simulink model "MRC_OutputMeasurement"  (R2016b)
settings: Solver=VariableStepAuto  StartTime=0.0  StopTime=10.0  RelTol=1e-3
undefined symbols (not defined in the file or in its folder): sigbuilder_block
settings Model: Creator=Niels  LastModifiedBy=Niels

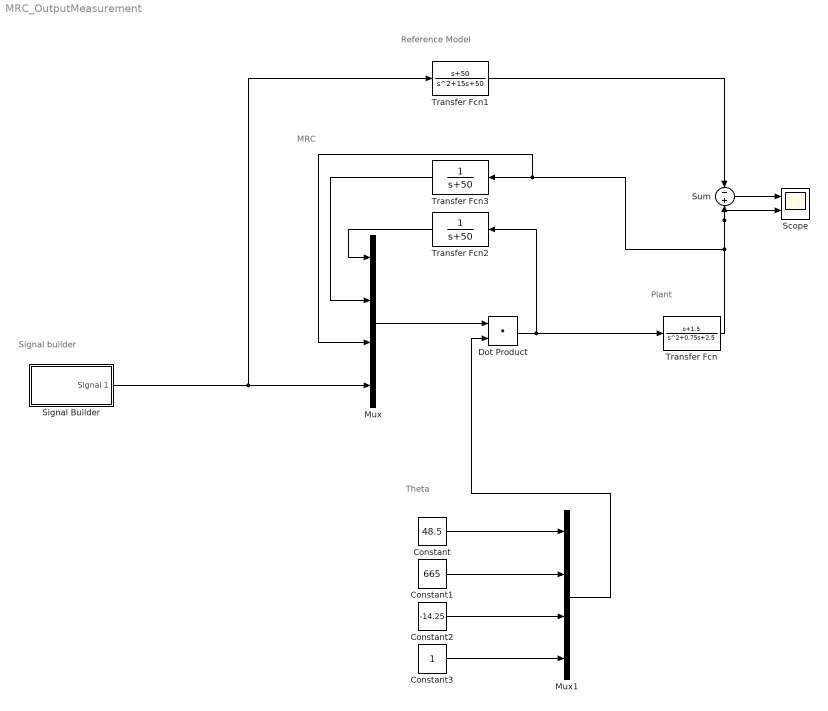
== system MRC_OutputMeasurement ==
  note: Signal builder
  note: Theta
  note: MRC
  note: Plant
  note: Reference Model
  Constant : Constant  Value=48.5
  Constant1 : Constant  Value=665
  Constant2 : Constant  Value=-14.25
  Constant3 : Constant
  Dot Product : DotProduct  InputSameDT=on  OutDataTypeStr=Inherit: Inherit via internal rule
  Mux : Mux
  Mux1 : Mux
  Scope : Scope  NumInputPorts=2
  Signal Builder : Subsystem  Tag=STV Subsys  LoadFcn=sigbuilder_block('load');  StartFcn=sigbuilder_block('start');  StopFcn=sigbuilder_block('stop');  ClipboardFcn=sigbuilder_block('clipboard');  mask(Sigbuilder block){tuvar=[0:10]}
      mask help: Simulink:masks:SigbuilderBlock_MD
      mask init:
      | if ~strcmp(get_param(bdroot(gcbh),'SimulationStatus'),'stopped') tuvar = sigbuilder_block('maskInit'); end
      settings: CopyFcn=sigbuilder_block('copy');  DeleteFcn=sigbuilder_block('delete');  ModelCloseFcn=sigbuilder_block('modelClose');  PreSaveFcn=sigbuilder_block('preSave');  PauseFcn=sigbuilder_block('pause');  ContinueFcn=sigbuilder_block('continue');  NameChangeFcn=sigbuilder_block('namechange');  OpenFcn=sigbuilder_block('open',[437.6 199.2 550.4 400 ]);  CloseFcn=sigbuilder_block('close');
      mask Display: plot(0, 0, 100, 100,[2, 2, 32, 32, 2], [68, 8, 8, 68, 68],[32, 2], [38, 38], [32, 19, 2],[53, 60, 44], [32, 17, 17, 2],[16, 16, 31, 31]);txt = getActiveGroup(gcbh);text(2, 100, txt,'verticalAlignment', 'top');
  Sum : Sum  Inputs=-|+
  Transfer Fcn : TransferFcn  Numerator=[1 1.5]  Denominator=[1 0.75 2.5]  ContinuousStateAttributes='Yp'
  Transfer Fcn1 : TransferFcn  Numerator=[1 50]  Denominator=[1 15 50]
  Transfer Fcn2 : TransferFcn  Denominator=[1 50]
  Transfer Fcn3 : TransferFcn  Denominator=[1 50]
  wires:
  Signal Builder/1(Signal 1) -> Transfer Fcn1/1, Mux/4
  Mux/1 -> Dot Product/1
  Dot Product/1 -> Transfer Fcn2/1, Transfer Fcn/1
  Transfer Fcn1/1 -> Sum/1
  Transfer Fcn/1 -> Mux/3, Transfer Fcn3/1, Scope/2, Sum/2
  Sum/1 -> Scope/1
  Constant/1 -> Mux1/1
  Constant1/1 -> Mux1/2
  Constant2/1 -> Mux1/3
  Constant3/1 -> Mux1/4
  Mux1/1 -> Dot Product/2
  Transfer Fcn3/1 -> Mux/2
  Transfer Fcn2/1 -> Mux/1

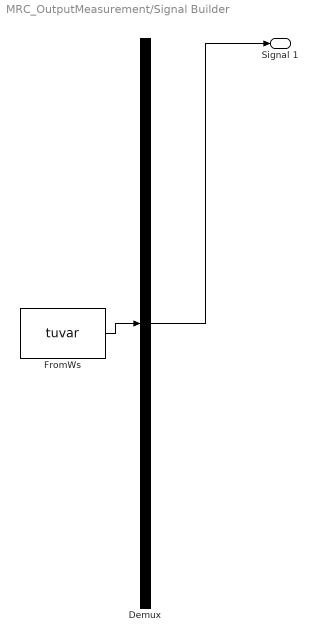
== system MRC_OutputMeasurement/Signal Builder ==
  Demux : Demux  Tag=STV Demux  Outputs=1
  FromWs : FromWorkspace  Tag=STV FromWs  VariableName=tuvar  SampleTime=0
      SigBuilderData=|
      | common.afterFinalStr = 'Extrapolate'
      | common.sampleTime = 0
      | dataSet.timeRange = [0 10]
      | dataSet.name = 'Group 1'
      | sbobj.Groups.Name = 'Group 1'
      | sbobj.Groups.Signals.Name = 'Signal 1'
      | sbobj.Groups.Signals.XData = [0 1.48 1.48 10]
      | sbobj.Groups.Signals.YData = [0 0 1 1]
  Signal 1 : Outport  Tag=STV Outport
  wires:
  Demux/1 -> Signal 1/1
  FromWs/1 -> Demux/1
